simulink model "read_state"  (R2020a)
settings: Solver=FixedStepDiscrete  StartTime=0.0  StopTime=10.0  RelTol=1e-3
settings Model: Creator=thomas  LastModifiedBy=thomas

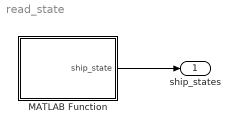
== system read_state ==
  MATLAB Function : MATLAB Function  TreatAsAtomicUnit=on
  ship_states : Outport  OutDataTypeStr=Bus: ShipStates
  wires:
  MATLAB Function/1(ship_state) -> ship_states/1

== matlab function read_state/MATLAB Function ==
  data: ship_state output Bus: ShipStates
function ship_state =read_state
    coder.extrinsic('evalin');
    ship_state.SAS = false;
    ship_state.RCS = false;
    ship_state.throttle = 1.0;
    ship_state.SAS = evalin('base', 'vessel_control.getSAS();');
    ship_state.RCS = evalin('base', 'vessel_control.getRCS();');
    ship_state.throttle = evalin('base', 'vessel_control.getThrottle();');
    evalin('base', 'AAtmp = vessel_flight.getRotation();');
    ship_state.rotation = zeros(1,4);
    ship_state.rotation(1) = evalin('base', 'AAtmp.getValue(3);');
    ship_state.rotation(2) = evalin('base', 'AAtmp.getValue(0);');
    ship_state.rotation(3) = evalin('base', 'AAtmp.getValue(1);');
    ship_state.rotation(4) = evalin('base', 'AAtmp.getValue(2);');
    ship_state.thrust = evalin('base', 'vessel.getThrust();');
    ship_state.sea_altitude = evalin('base', 'vessel_flight.getMeanAltitude();');
    evalin('base', 'tmpVelocity = vessel_flight.getVelocity();');
    ship_state.velocity = zeros(3,1);
    ship_state.velocity(1) = evalin('base', 'tmpVelocity.getValue(0);');
    ship_state.velocity(2) = evalin('base', 'tmpVelocity.getValue(1);');
    ship_state.velocity(3) = evalin('base', 'tmpVelocity.getValue(2);');
    ship_state.pitch = evalin('base', 'vessel_flight.getPitch();');
    ship_state.yaw = evalin('base', 'vessel_flight.getHeading();');
    ship_state.roll = evalin('base', 'vessel_flight.getRoll();');
    ship_state.atmosphere_density = evalin('base', 'vessel_flight.getAtmosphereDensity();');
    ship_state.dynamic_pressure = evalin('base', 'vessel_flight.getDynamicPressure();');
    ship_state.static_pressure = evalin('base', 'vessel_flight.getStaticPressure();');
    evalin('base', 'tmp = vessel.angularVelocity(vessel_surface_rf);');
    ship_state.angular_velocity_surface = zeros(3,1);
    ship_state.angular_velocity_surface(1) = evalin('base', 'tmp.getValue(0);');
    ship_state.angular_velocity_surface(2) = evalin('base', 'tmp.getValue(1);');
    ship_state.angular_velocity_surface(3) = evalin('base', 'tmp.getValue(2);');
    
end
